simulink model "filtro_LP_corriente"  (R2021a)
settings: Solver=VariableStepAuto  StartTime=0.0  StopTime=10.0  RelTol=1e-3
undefined symbols (not defined in the file): wn_i
settings Model: Creator=fhlla  LastModifiedBy=fhlla

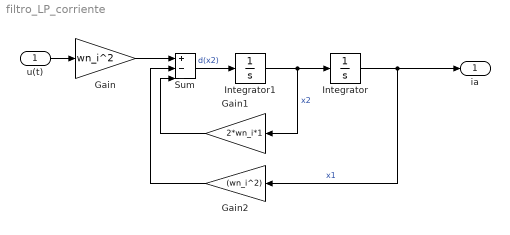
== system filtro_LP_corriente ==
  u(t) : Inport
  Gain : Gain  Gain=wn_i^2
  Gain1 : Gain  Gain=2*wn_i*1
  Gain2 : Gain  Gain=(wn_i^2)
  Integrator : Integrator
  Integrator1 : Integrator
  Sum : Sum  Inputs=|+|-|-
  ia : Outport
  wires:
  Integrator1/1 -> Gain1/1, Integrator/1  "x2"
  Gain2/1 -> Sum/2
  Integrator/1 -> Gain2/1, ia/1  "x1"
  Gain/1 -> Sum/1
  Sum/1 -> Integrator1/1  "d(x2)"
  Gain1/1 -> Sum/3
  u(t)/1 -> Gain/1
